simulink model "schema"  (R2016a)
settings: Solver=VariableStepAuto  StartTime=0.0  StopTime=10.0  RelTol=1e-3
values from neighbouring files (symbols this model uses):
  Ts = 0.05    [model.m]
  x10_0 = 0    [model.m]
  x11_0 = 0    [model.m]
  x12_0 = 0    [model.m]
  x1_0 = 0    [model.m]
  x2_0 = 0    [model.m]
  x3_0 = 0    [model.m]
  x4_0 = 0    [model.m]
  x5_0 = 0    [model.m]
  x6_0 = 0    [model.m]
  x7_0 = 0    [model.m]
  x8_0 = 0    [model.m]
  x9_0 = 0    [model.m]
undefined symbols (not defined in the file or in its folder): A, B, C, D
libraries: mpclib x1
settings Model: Creator=37544  LastModifiedBy=37544

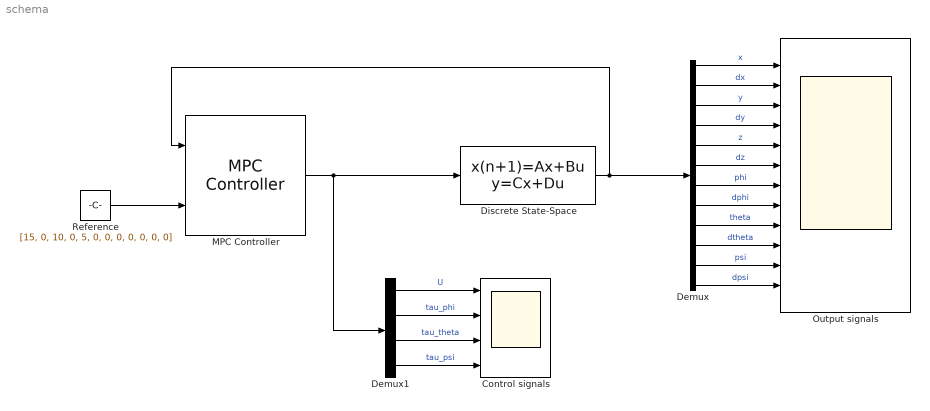
== system schema ==
  "Control signals " : Scope  NumInputPorts=4
  Demux : Demux  Outputs=12
  Demux1 : Demux
  Discrete State-Space : DiscreteStateSpace  A=A  B=B  C=C  D=D  X0=[x1_0,x2_0,x3_0,x4_0,x5_0,x6_0,x7_0,x8_0,x9_0,x10_0,x11_0,x12_0]  SampleTime=Ts
  MPC Controller : mpclib/MPC Controller  SCDEnableBlockLinearizationSpecification=on  mpcobj=mpc1  is_multiple=0  enable_value=0  return_u0=off  ref_from_ws=off  ref_signal_name=[]  ref_preview=off  md_from_ws=off  md_signal_name=[]  md_preview=off  from_project=off  project_file=MPCtask.mat  md_inport=off  mv_inport=off  cost_outport=off  return_sequence=off  return_qpstatus=off  return_state=off  state_inport=off  lims_inport=off  ywt_inport=off  is_designfromscratch=0  uwt_inport=off  duwt_inport=off  rhoeps_inport=off  uref_inport=off  n_ts=0.05  n_mv=4  n_md=0  n_ud=0  n_mo=12  n_uo=0  BlockDataType=double  SampleTimeInherited=off  switch_inport=off
  "Output signals " : Scope  NumInputPorts=12
  "Reference " : Constant  Value=[15, 0, 10, 0, 5, 0, 0, 0, 0, 0, 0, 0]  SampleTime=Ts
  wires:
  MPC Controller/1 -> Discrete State-Space/1, Demux1/1
  Discrete State-Space/1 -> MPC Controller/1, Demux/1
  "Reference "/1 -> MPC Controller/2
  Demux/1 -> "Output signals "/1  "x"
  Demux/2 -> "Output signals "/2  "dx"
  Demux/3 -> "Output signals "/3  "y"
  Demux/4 -> "Output signals "/4  "dy"
  Demux/5 -> "Output signals "/5  "z"
  Demux/6 -> "Output signals "/6  "dz"
  Demux/7 -> "Output signals "/7  "phi"
  Demux/8 -> "Output signals "/8  "dphi"
  Demux/9 -> "Output signals "/9  "theta"
  Demux/10 -> "Output signals "/10  "dtheta"
  Demux/11 -> "Output signals "/11  "psi"
  Demux/12 -> "Output signals "/12  "dpsi"
  Demux1/1 -> "Control signals "/1  "U"
  Demux1/2 -> "Control signals "/2  "tau_phi"
  Demux1/3 -> "Control signals "/3  "tau_theta"
  Demux1/4 -> "Control signals "/4  "tau_psi"
